simulink model "sim_pos_control_pid"  (R2020b)
settings: Solver=ode1  StartTime=0.0  StopTime=200  FixedStep=0.01  RelTol=1e-3
values from neighbouring files (symbols this model uses):
  a = 27.65    [parameter.m]
  b = 17.35    [parameter.m]
  Kd = (2*zeta*wn + lamda_1 -a)/b    (= 0.784244211034)    [parameter.m]
  Ki = (wn^2*lamda_1)/b    (= 0.910165247363)    [parameter.m]
  Kp = (2*zeta*wn*lamda_1 + wn^2)/b    (= 2.91990009415)    [parameter.m]
settings Model: Creator=ONLY-GOD  LastModifiedBy=ONLY-GOD

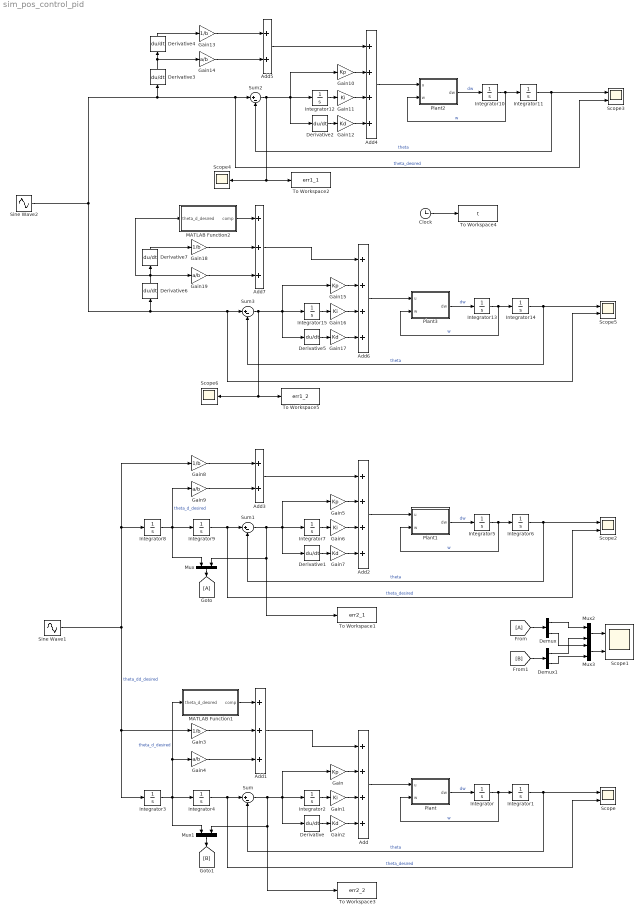
== system sim_pos_control_pid ==
  Add{,2,4,6} (4 alike) : Sum  Inputs=++++
  Add1 : Sum  Inputs=+++
  Add3 : Sum
  Add5 : Sum
  Add7 : Sum  Inputs=+++
  Clock : Clock
  Demux : Demux  Outputs=2
  Demux1 : Demux  Outputs=2
  Derivative{,1..7} (8 alike) : Derivative
  Gain{,5,10,15} (4 alike) : Gain  Gain=Kp
  Gain{1,6,11,16} (4 alike) : Gain  Gain=Ki
  Gain{2,7,12,17} (4 alike) : Gain  Gain=Kd
  Gain{3,8,13,18} (4 alike) : Gain  Gain=1/b
  Gain{4,9,14,19} (4 alike) : Gain  Gain=a/b
  Integrator{,1..15} (16 alike) : Integrator
  MATLAB Function1 : MATLAB Function  TreatAsAtomicUnit=on
  MATLAB Function2 : MATLAB Function  TreatAsAtomicUnit=on
  Mux{,1..3} (4 alike) : Mux  Inputs=2
  Plant : MATLAB Function  TreatAsAtomicUnit=on
  Plant1 : MATLAB Function  TreatAsAtomicUnit=on
  Plant2 : MATLAB Function  TreatAsAtomicUnit=on
  Plant3 : MATLAB Function  TreatAsAtomicUnit=on
  Scope{,1..3,5} (5 alike) : Scope  NumInputPorts=2
  Scope4 : Scope
  Scope6 : Scope
  Sine Wave1 : Sin  Amplitude=10  Frequency=2*pi*0.1  SampleTime=0
  Sine Wave2 : Sin  Amplitude=20  Frequency=2*pi*0.1  SampleTime=0
  Sum{,1..3} (4 alike) : Sum  Inputs=|+-
  To Workspace1 : ToWorkspace  VariableName=err2_1  SampleTime=-1
      settings: Save2DSignal=2-D array (concatenate along first dimension)
  To Workspace2 : ToWorkspace  VariableName=err1_1  SampleTime=-1
      settings: Save2DSignal=2-D array (concatenate along first dimension)
  To Workspace3 : ToWorkspace  VariableName=err2_2  SampleTime=-1
      settings: Save2DSignal=2-D array (concatenate along first dimension)
  To Workspace4 : ToWorkspace  VariableName=t  SampleTime=-1
      settings: Save2DSignal=2-D array (concatenate along first dimension)
  To Workspace5 : ToWorkspace  VariableName=err1_2  SampleTime=-1
      settings: Save2DSignal=2-D array (concatenate along first dimension)
  wires:
  Integrator/1 -> Plant/2(w), Integrator1/1  "w"
  Sum/1 -> Mux1/2, To Workspace3/1, Derivative/1, Integrator2/1, Gain/1
  Plant/1(dw) -> Integrator/1  "dw"
  Derivative/1 -> Gain2/1
  Integrator2/1 -> Gain1/1
  Gain/1 -> Add/2
  Gain2/1 -> Add/4
  Gain1/1 -> Add/3
  Add/1 -> Plant/1(u)
  Add1/1 -> Add/1
  Gain3/1 -> Add1/2
  Gain4/1 -> Add1/3
  Sine Wave1/1 -> Integrator8/1, Gain8/1, Gain3/1, Integrator3/1  "theta_dd_desired"
  Integrator3/1 -> Mux1/1, MATLAB Function1/1(theta_d_desired), Gain4/1, Integrator4/1  "theta_d_desired"
  MATLAB Function1/1(comp) -> Add1/1
  Integrator9/1 -> Sum1/1, Scope2/2  "theta_desired"
  Integrator8/1 -> Mux/1, Integrator9/1, Gain9/1  "theta_d_desired"
  Gain9/1 -> Add3/2
  Gain8/1 -> Add3/1
  Add3/1 -> Add2/1
  Add2/1 -> Plant1/1(u)
  Gain6/1 -> Add2/3
  Gain7/1 -> Add2/4
  Gain5/1 -> Add2/2
  Integrator7/1 -> Gain6/1
  Derivative1/1 -> Gain7/1
  Plant1/1(dw) -> Integrator5/1  "dw"
  Sum1/1 -> Mux/2, To Workspace1/1, Gain5/1, Integrator7/1, Derivative1/1
  Integrator5/1 -> Integrator6/1, Plant1/2(w)  "w"
  Integrator6/1 -> Sum1/2, Scope2/1  "theta"
  Mux/1 -> [A]
  Mux1/1 -> [B]
  [B] -> Demux1/1
  [A] -> Demux/1
  Mux2/1 -> Scope1/1
  Mux3/1 -> Scope1/2
  Demux/1 -> Mux2/1
  Demux1/1 -> Mux2/2
  Demux/2 -> Mux3/1
  Demux1/2 -> Mux3/2
  Integrator11/1 -> Scope3/1, Sum2/2  "theta"
  Integrator10/1 -> Plant2/2(w), Integrator11/1  "w"
  Sum2/1 -> To Workspace2/1, Scope4/1, Derivative2/1, Integrator12/1, Gain10/1
  Plant2/1(dw) -> Integrator10/1  "dw"
  Derivative2/1 -> Gain12/1
  Integrator12/1 -> Gain11/1
  Gain10/1 -> Add4/2
  Gain12/1 -> Add4/4
  Gain11/1 -> Add4/3
  Add4/1 -> Plant2/1(u)
  Add5/1 -> Add4/1
  Gain13/1 -> Add5/1
  Gain14/1 -> Add5/2
  Derivative3/1 -> Derivative4/1, Gain14/1
  Derivative4/1 -> Gain13/1
  Integrator1/1 -> Scope/1, Sum/2  "theta"
  Integrator4/1 -> Scope/2, Sum/1  "theta_desired"
  Clock/1 -> To Workspace4/1
  Derivative7/1 -> Gain18/1
  Derivative6/1 -> Gain19/1, MATLAB Function2/1(theta_d_desired), Derivative7/1
  Sine Wave2/1 -> Scope3/2, Sum2/1, Derivative3/1, Derivative6/1, Sum3/1, Scope5/2  "theta_desired"
  Gain19/1 -> Add7/3
  Gain18/1 -> Add7/2
  Add7/1 -> Add6/1
  Add6/1 -> Plant3/1(u)
  Gain16/1 -> Add6/3
  Gain17/1 -> Add6/4
  Gain15/1 -> Add6/2
  Integrator15/1 -> Gain16/1
  Derivative5/1 -> Gain17/1
  Plant3/1(dw) -> Integrator13/1  "dw"
  Sum3/1 -> Gain15/1, Integrator15/1, Derivative5/1, To Workspace5/1, Scope6/1
  Integrator13/1 -> Integrator14/1, Plant3/2(w)  "w"
  Integrator14/1 -> Sum3/2, Scope5/1  "theta"
  MATLAB Function2/1(comp) -> Add7/1

== matlab function sim_pos_control_pid/Plant ==
  settings: updateMethod=DISCRETE
  data: u input; dw output; w input
function dw = dcmotor(u,w)

a = 27.65; b = 17.35; c = 5.63;
dw = -a*w+b*u-c*sign(w) + 1e-4*randn;

== matlab function sim_pos_control_pid/Plant2 ==
  settings: updateMethod=DISCRETE
  data: u input; dw output; w input
function dw = dcmotor(u,w)

a = 27.65; b = 17.35; c = 5.63;
dw = -a*w+b*u-c*sign(w) + 1e-4*randn;

== matlab function sim_pos_control_pid/Plant1 ==
  settings: updateMethod=DISCRETE
  data: u input; dw output; w input
function dw = dcmotor(u,w)

a = 27.65; b = 17.35; c = 5.63;
dw = -a*w+b*u-c*sign(w) + 1e-4*randn;

== matlab function sim_pos_control_pid/Plant3 ==
  settings: updateMethod=DISCRETE
  data: u input; dw output; w input
function dw = dcmotor(u,w)

a = 27.65; b = 17.35; c = 5.63;
dw = -a*w+b*u-c*sign(w) + 1e-4*randn;

== matlab function sim_pos_control_pid/MATLAB Function2 ==
  settings: updateMethod=DISCRETE
  data: theta_d_desired input; comp output
function comp = fcn(theta_d_desired)

b = 17.35; c = 5.63; %+ 0.3*rand;
comp = c/b*sign(theta_d_desired);

== matlab function sim_pos_control_pid/MATLAB Function1 ==
  settings: updateMethod=DISCRETE
  data: theta_d_desired input; comp output
function comp = fcn(theta_d_desired)

b = 17.35; c = 5.63; %+ 0.3*rand;
comp = c/b*sign(theta_d_desired);
